simulink model "comparison"  (Simulink 7.9)
settings: Solver=ode45  StartTime=0.0  StopTime=20  RelTol=1e-3
values from neighbouring files (symbols this model uses):
  d1bar = 0    [script.m]
  d2bar = 0    [script.m]
  Ibar = sign(wbar)*Ifr + b*abs(wbar)*wbar/K + d1bar    [script.m]
  Ubar = R*Ibar+K*wbar-d2bar    [script.m]
  wbar = 300    [script.m]
undefined symbols (not defined in the file or in its folder): syss
libraries: cstblocks x1, simulink x1
settings Model: Creator=PhM  LastModifiedBy=PhM
settings OptimizationCC: InitFltsAndDblsToZero=on
settings DebuggingCC: SaveWithParameterizedLinksMsg=none  SignalResolutionControl=TryResolveAllWithWarning  MultiTaskDSMMsg=warning  MultiTaskCondExecSysMsg=none  FcnCallInpInsideContextMsg=Use local settings  StrictBusMsg=None
settings RTWCC: IncludeERTFirstTime=on
settings GRTTargetCC: TargetFcnLib=ansi_tfl_tmw.mat  CombineOutputUpdateFcns=off  GRTInterface=on

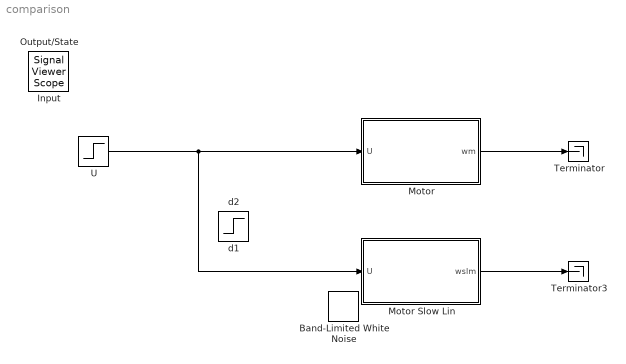
== system comparison ==
  Motor : Subsystem
  Motor Slow Lin : Subsystem
  Terminator : Terminator
  Terminator3 : Terminator
  U : Step  Time=5  Before=Ubar  After=Ubar+1  SampleTime=0
  Band-Limited White Noise : simulink/Sources/Band-Limited White Noise  IOType=siggen  Cov=1e-2  Ts=1e-2  seed=[23341]
  Input : SignalViewerScope  IOType=viewer  NumInputPorts=3  LegendLocations=|  RefreshTime=0.035000
      | 0.72967      0.9209     0.20122    0.028719
      |   0.719     0.60805     0.21341    0.028719
      |   0.719     0.29732     0.21341    0.028719
      settings: ShowLegends=on  TimeRange=20  YMin=4.5~0~0  YMax=6.000000000000001~1~1
  Output/State : SignalViewerScope  IOType=viewer  NumInputPorts=3  RefreshTime=0.035000
      settings: TimeRange=20  YMin=290~300~2  YMax=380~380~5.5
  d1 : Step  IOType=siggen  Time=10  Before=d1bar  After=d1bar+1  SampleTime=0
  d2 : Step  IOType=siggen  Time=15  Before=d2bar  After=d2bar+1  SampleTime=0
  wires:
  Motor/1(wm) -> Terminator/1
  U/1 -> Motor/1(U), Motor Slow Lin/1(U)
  Motor Slow Lin/1(wslm) -> Terminator3/1

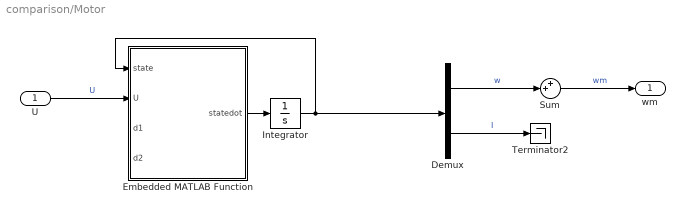
== system comparison/Motor ==
  U : Inport
  Demux : Demux  Outputs=2
  Embedded MATLAB Function : MATLAB Function  TreatAsAtomicUnit=on
  Integrator : Integrator  InitialCondition=[wbar; Ibar]
  Sum : Sum  Inputs=++|
  Terminator2 : Terminator
  wm : Outport
  wires:
  Embedded MATLAB Function/1(statedot) -> Integrator/1
  Integrator/1 -> Embedded MATLAB Function/1(state), Demux/1
  Demux/1 -> Sum/2  "w"
  Demux/2 -> Terminator2/1  "I"
  U/1 -> Embedded MATLAB Function/2(U)  "U"
  Sum/1 -> wm/1  "wm"

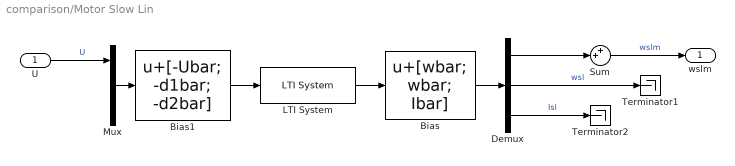
== system comparison/Motor Slow Lin ==
  U : Inport
  Bias : Bias  Bias=[wbar; wbar; Ibar]
  Bias1 : Bias  Bias=[-Ubar; -d1bar; -d2bar]
  Demux : Demux  Outputs=3
  LTI System : cstblocks/LTI System  sys=syss(:,:,2)  IC=0
  Mux : Mux  Inputs=3
  Sum : Sum  Inputs=++|
  Terminator1 : Terminator
  Terminator2 : Terminator
  wslm : Outport
  wires:
  Bias1/1 -> LTI System/1
  Bias/1 -> Demux/1
  LTI System/1 -> Bias/1
  Mux/1 -> Bias1/1
  U/1 -> Mux/1  "U"
  Demux/1 -> Sum/2
  Demux/2 -> Terminator1/1  "wsl"
  Demux/3 -> Terminator2/1  "Isl"
  Sum/1 -> wslm/1  "wslm"

== matlab function Motor/Embedded MATLAB Function ==
  data: state input double; statedot output double; U input double; d1 input double; d2 input double
function statedot = fcn(state,U,d1,d2)
% This block supports an embeddable subset of the MATLAB language.
% See the help menu for details. 

R = 0.56;
L = 4e-3;
Ifr = 0.4;
K = 1.19e-2;
J = 3.45e-5;
b = 2.4e-7;

w = state(1);
I = state(2);

wdot = (K*I  - sign(w)*K*Ifr - b*abs(w)*w - K*d1)/J;
Idot = (-R*I-K*w+U+d2)/L;

statedot = [wdot; Idot];
